simulink model "Lab_1_Part_1_2"  (R2019b)
settings: Solver=VariableStepAuto  StartTime=0.0  StopTime=10.0  RelTol=1e-3
libraries: powerlib_meascontrol x2
settings Model: Creator=mikewang  LastModifiedBy=mikewang

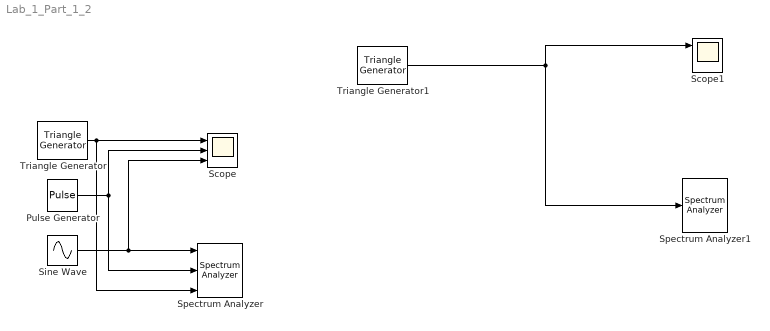
== system Lab_1_Part_1_2 ==
  Pulse Generator : DiscretePulseGenerator  Period=100  PulseWidth=5  SampleTime=1e-6
  Scope : Scope  NumInputPorts=3
  Scope1 : Scope  NumInputPorts=3
  Sine Wave : Sin  SineType=Sample based  Samples=100  SampleTime=1e-6
  Spectrum Analyzer : SpectrumAnalyzer  NumInputPorts=3
  Spectrum Analyzer1 : SpectrumAnalyzer  NumInputPorts=3
  Triangle Generator : powerlib_meascontrol/Pulse & Signal Generators/Triangle Generator  Freq=1e3  Phase=90  Ts=1e-6
      settings: SourceProductName=Simscape Electrical
  Triangle Generator1 : powerlib_meascontrol/Pulse & Signal Generators/Triangle Generator  Freq=1e4  Phase=90  Ts=1e-6
      settings: SourceProductName=Simscape Electrical
  wires:
  Triangle Generator/1 -> Spectrum Analyzer/3, Scope/1
  Pulse Generator/1 -> Spectrum Analyzer/2, Scope/2
  Sine Wave/1 -> Spectrum Analyzer/1, Scope/3
  Triangle Generator1/1 -> Scope1/1, Spectrum Analyzer1/2
